simulink model "kal3slx"  (R2019b)
settings: Solver=VariableStepAuto  StartTime=0.0  StopTime=10.0  RelTol=1e-3
libraries: simulink x2
settings Model: Creator=kWX1197707  LastModifiedBy=kWX1197707

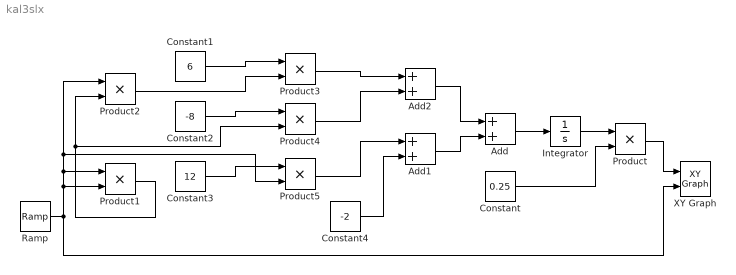
== system kal3slx ==
  Add : Sum
  Add1 : Sum
  Add2 : Sum
  Constant : Constant  Value=0.25
  Constant1 : Constant  Value=6
  Constant2 : Constant  Value=-8
  Constant3 : Constant  Value=12
  Constant4 : Constant  Value=-2
  Integrator : Integrator
  Product{,1..5} (6 alike) : Product
  Ramp : simulink/Sources/Ramp  slope=1  start=0  InitialOutput=0
  XY Graph : simulink/Sinks/XY Graph  xmin=-1  xmax=1  ymin=-1  ymax=1  st=-1
  wires:
  Integrator/1 -> Product/1
  Constant/1 -> Product/2
  Add/1 -> Integrator/1
  Add2/1 -> Add/1
  Add1/1 -> Add/2
  Ramp/1 -> XY Graph/2, Product1/2, Product1/1, Product5/2, Product2/1
  Product1/1 -> Product4/2, Product2/2
  Constant1/1 -> Product3/1
  Product2/1 -> Product3/2
  Constant2/1 -> Product4/1
  Constant3/1 -> Product5/1
  Product3/1 -> Add2/1
  Product4/1 -> Add2/2
  Product5/1 -> Add1/1
  Constant4/1 -> Add1/2
  Product/1 -> XY Graph/1
